simulink model "sampleModel1567_5_sub"  (R2023a)
settings: Solver=VariableStepAuto  StartTime=0.0  StopTime=10.0  RelTol=1e-3
libraries: hdlsllib x6
settings Model: Creator=user1  LastModifiedBy=user1

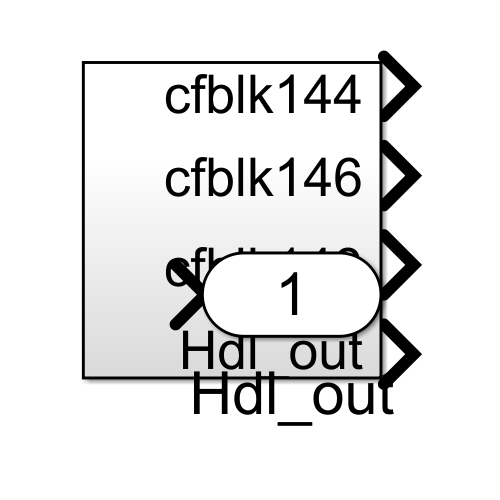
[thumbnail: Simulink's stored preview of the top-level diagram]
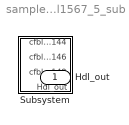
== system sampleModel1567_5_sub ==
  Subsystem : Subsystem
  Hdl_out : Outport  OutDataTypeStr=uint8

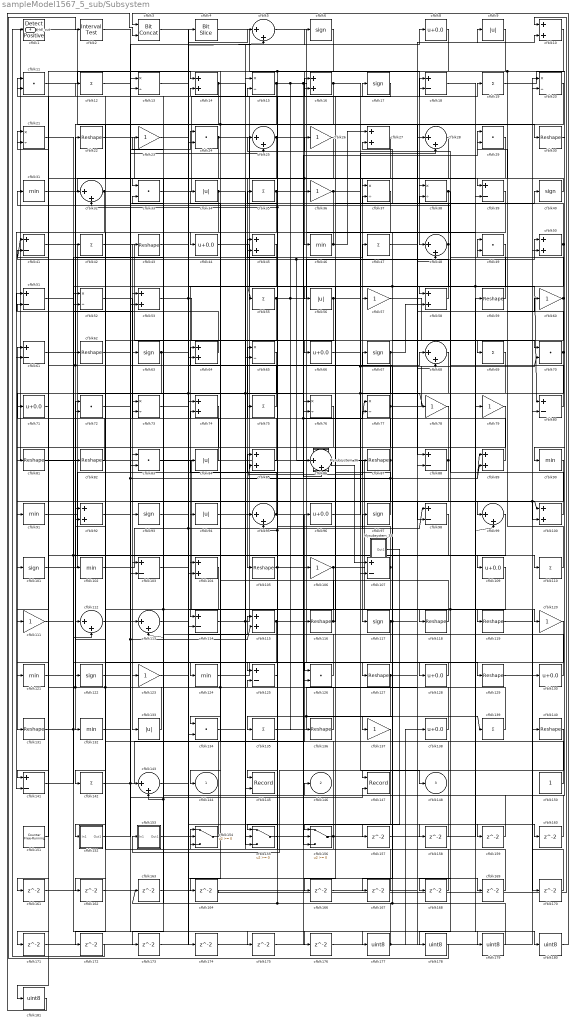
== system sampleModel1567_5_sub/Subsystem ==
  Mysubsystem_35 : Subsystem  TreatAsAtomicUnit=on  RTWFcnName=Mysubsystem_35
      settings: RTWFcnNameOpts=User specified  RTWFileNameOpts=Use function name
  Mysubsystem_36 : Subsystem  TreatAsAtomicUnit=on  RTWFcnName=Mysubsystem_36
      settings: RTWFcnNameOpts=User specified  RTWFileNameOpts=Use function name
  cfblk1 : hdlsllib/Logic and Bit Operations/Detect Rise Positive  vinit=0  OutDataTypeStr=uint8
  cfblk{10,14,16,27,45,50,53,58,64,74,85,89,92,100,104,115} (16 alike) : Sum  OutDataTypeStr=uint8
  cfblk{6,17,40,63,67,93,97,101,117,122} (10 alike) : Signum
  cfblk{31,46,90..91,102,121,124,132} (8 alike) : MinMax  OutDataTypeStr=uint8
  cfblk{18,39,41,51,61,80,88,98,103,107,114,125,141} (13 alike) : Sum  Inputs=+-  OutDataTypeStr=uint8
  cfblk{22,30,43,59,62,81..82,87,105,116,118..119,127,129,131,136,140} (17 alike) : Reshape
  cfblk{23,26,36,57,60,78..79,106,111,120,123,137} (12 alike) : Gain  OutDataTypeStr=uint8
  cfblk{8,44,66,71,96,109,128,130,138} (9 alike) : Bias  Bias=0.0  SaturateOnIntegerOverflow=off
  cfblk{11,24,29,33,49,70,72,83,126,134} (10 alike) : DotProduct  OutDataTypeStr=uint8
  cfblk{12,19,35,42,47,55,69,75,110,135,139,142} (12 alike) : Sum  Inputs=+  OutDataTypeStr=uint8
  cfblk{5,25,28,32,48,68,86,95,99,112..113,143} (12 alike) : Sum  Inputs=|++  OutDataTypeStr=uint8
  cfblk{13,15,20..21,37..38,52,65,73,76..77} (11 alike) : Product  Inputs=*/  OutDataTypeStr=uint8  RndMeth=Zero  SaturateOnIntegerOverflow=on
  cfblk{9,34,56,84,94,133} (6 alike) : Abs  OutDataTypeStr=uint8  SaturateOnIntegerOverflow=off
  cfblk145 : Record  FileSettingsInternal="{\"entries\":[{\"content\":{\"excelSettings\":{\"content\":{},\"type\":\"Streamout.ExcelSettings\"}},\"type\":\"Streamout.FileSettingStorage\",\"uuid\":\"\"}],\"packageUris\":[\"http:\\/\\/schema.mathworks.com\\/mf0\\/streamout_blocks\\/R2020a\"],\"version\":\"1.0\"}"  Layout=[1 1]  SignalsInternal="{\"entries\":[{\"content\":{\"signals\":[{\"content\":{\"blockPath\":[],\"dimensions\":[1],\"domain\":\"\",\"lineColor\":\"#a2142f\",\"plots\":[1],\"port\":1,\"signalID\":25340,\"signalName\":\"cfblk105\"},\"type\":\"RecordBlkView.Signal\",\"uuid\":\"\"},{\"content\":{\"blockPath\":[],\"dimensions\":[1],\"domain\":\"\",\"lineColor\":\"#139fff\",\"plots\":[1],\"port\":2,\"signalID\":25343,\"signalName\":\"cfblk109\"},\"type\":\"RecordBlkView.Signal\",\"uuid\":\"\"}]},\"type\":\"RecordBlkView.InputSignals\",\"uuid\":\"\"}],\"packageUris\":[\"http:\\/\\/schema.mathworks.com\\/mf0\\/streamout_blocks\\/R2020a\"],\"version\":\"1.0\"}"  VisualizationBindings="{\"xyplotplugin\":{\"info\":[{\"series\":[{\"bindingParametersList\":[{\"parameter\":\"X-Axis\",\"signalID\":25340,\"signalName\":\"cfblk105\"},{\"parameter\":\"Y-Axis\",\"signalID\":25343,\"signalName\":\"cfblk109\"}],\"seriesID\":58215}],\"subplotID\":1}]}}"  CompatibilityTag=XY  st=-1
  cfblk147 : Record  FileSettingsInternal="{\"entries\":[{\"content\":{\"excelSettings\":{\"content\":{},\"type\":\"Streamout.ExcelSettings\"}},\"type\":\"Streamout.FileSettingStorage\",\"uuid\":\"\"}],\"packageUris\":[\"http:\\/\\/schema.mathworks.com\\/mf0\\/streamout_blocks\\/R2020a\"],\"version\":\"1.0\"}"  Layout=[1 1]  SignalsInternal="{\"entries\":[{\"content\":{\"signals\":[{\"content\":{\"blockPath\":[],\"dimensions\":[1],\"domain\":\"\",\"lineColor\":\"#a2142f\",\"plots\":[1],\"port\":1,\"signalID\":25332,\"signalName\":\"cfblk117\"},\"type\":\"RecordBlkView.Signal\",\"uuid\":\"\"},{\"content\":{\"blockPath\":[],\"dimensions\":[1],\"domain\":\"\",\"lineColor\":\"#139fff\",\"plots\":[1],\"port\":2,\"signalID\":25335,\"signalName\":\"cfblk142\"},\"type\":\"RecordBlkView.Signal\",\"uuid\":\"\"}]},\"type\":\"RecordBlkView.InputSignals\",\"uuid\":\"\"}],\"packageUris\":[\"http:\\/\\/schema.mathworks.com\\/mf0\\/streamout_blocks\\/R2020a\"],\"version\":\"1.0\"}"  VisualizationBindings="{\"xyplotplugin\":{\"info\":[{\"series\":[{\"bindingParametersList\":[{\"parameter\":\"X-Axis\",\"signalID\":25332,\"signalName\":\"cfblk117\"},{\"parameter\":\"Y-Axis\",\"signalID\":25335,\"signalName\":\"cfblk142\"}],\"seriesID\":62710}],\"subplotID\":1}]}}"  CompatibilityTag=XY  st=-1
  cfblk150 : Constant  OutDataTypeStr=uint8  SampleTime=-1
  cfblk151 : hdlsllib/Sources/Counter Free-Running  NumBits=16  tsamp=-1
  cfblk152 : Subsystem
      settings: LibrarySourceBlock=|
      | hdlsllib/Ports &
      | Subsystems/Subsystem
  cfblk153 : Subsystem
      settings: LibrarySourceBlock=|
      | hdlsllib/Ports &
      | Subsystems/Subsystem
  cfblk154 : Switch  OutDataTypeStr=uint8  SaturateOnIntegerOverflow=off  InputSameDT=off
  cfblk155 : Switch  OutDataTypeStr=uint8  SaturateOnIntegerOverflow=off  InputSameDT=off
  cfblk156 : Switch  OutDataTypeStr=uint8  SaturateOnIntegerOverflow=off  InputSameDT=off
  cfblk{157..164,166..176} (19 alike) : Delay  SampleTime=1
  cfblk{177..181} (5 alike) : DataTypeConversion  OutDataTypeStr=uint8  SaturateOnIntegerOverflow=off  RndMeth=Floor
  cfblk2 : hdlsllib/Logic and Bit Operations/Interval Test  IntervalClosedRight=on  uplimit=0.5  IntervalClosedLeft=on  lowlimit=-0.5  OutDataTypeStr=uint8
  cfblk3 : hdlsllib/Logic and Bit Operations/Bit Concat  numInputs=2
  cfblk4 : hdlsllib/Logic and Bit Operations/Bit Slice  lidx=7  ridx=0
  cfblk144 : Outport  OutDataTypeStr=uint8  VectorParamsAs1DForOutWhenUnconnected=off
  cfblk146 : Outport  Port=2  OutDataTypeStr=uint8  VectorParamsAs1DForOutWhenUnconnected=off
  cfblk148 : Outport  Port=3  OutDataTypeStr=uint8  VectorParamsAs1DForOutWhenUnconnected=off
  Hdl_out : Outport  Port=4  OutDataTypeStr=uint8
  wires:
  cfblk40/1 -> cfblk33/1
  cfblk20/1 -> cfblk132/1
  cfblk56/1 -> cfblk58/1, cfblk142/1
  cfblk75/1 -> cfblk41/2, cfblk22/1
  cfblk107/1 -> cfblk133/1, cfblk32/2, cfblk11/2
  cfblk127/1 -> cfblk60/1, cfblk154/1
  cfblk63/1 -> cfblk5/1, cfblk131/1
  cfblk41/1 -> cfblk110/1
  cfblk140/1 -> cfblk153/1(In1)
  cfblk33/1 -> cfblk17/1
  cfblk153/1(Out1) -> cfblk98/1, cfblk4/1
  cfblk91/1 -> cfblk109/1
  cfblk44/1 -> cfblk99/2, cfblk80/1
  cfblk35/1 -> cfblk141/2, cfblk128/1
  cfblk114/1 -> cfblk8/1, cfblk19/1
  cfblk67/1 -> cfblk58/2, cfblk164/1, cfblk155/3
  cfblk59/1 -> cfblk31/1
  cfblk87/1 -> Hdl_out/1, cfblk12/1, cfblk114/1
  cfblk27/1 -> cfblk105/1
  cfblk22/1 -> cfblk117/1
  cfblk83/1 -> cfblk120/1
  cfblk136/1 -> cfblk11/1, cfblk72/1
  cfblk79/1 -> cfblk144/1
  cfblk84/1 -> cfblk61/1
  cfblk126/1 -> cfblk95/2, cfblk35/1
  cfblk99/1 -> cfblk122/1
  cfblk90/1 -> cfblk123/1
  cfblk42/1 -> cfblk69/1
  cfblk48/1 -> cfblk16/1, cfblk55/1, cfblk137/1
  cfblk8/1 -> cfblk46/1
  cfblk122/1 -> cfblk115/2, cfblk89/1, cfblk45/1
  cfblk5/1 -> cfblk79/1
  cfblk106/1 -> cfblk155/2, cfblk119/1
  cfblk69/1 -> cfblk93/1
  cfblk12/1 -> cfblk113/1
  cfblk19/1 -> cfblk146/1
  cfblk141/1 -> cfblk52/1
  cfblk15/1 -> cfblk106/1, cfblk39/2, cfblk30/1, cfblk32/1, cfblk124/1
  cfblk85/1 -> cfblk65/1
  cfblk142/1 -> cfblk147/2, cfblk96/1
  cfblk46/1 -> cfblk27/1, cfblk44/1
  cfblk50/1 -> cfblk27/2, cfblk94/1
  cfblk53/1 -> cfblk5/2, cfblk66/1
  cfblk81/1 -> cfblk82/1
  cfblk25/1 -> cfblk171/1, cfblk37/1
  cfblk86/1 -> cfblk140/1
  cfblk29/1 -> cfblk36/1, cfblk173/1, cfblk143/2
  cfblk89/1 -> cfblk43/1
  cfblk131/1 -> cfblk176/1, cfblk47/1
  cfblk113/1 -> cfblk74/1
  cfblk130/1 -> cfblk42/1
  cfblk150/1 -> cfblk74/2
  cfblk4/1 -> cfblk48/1
  cfblk57/1 -> cfblk70/1
  cfblk9/1 -> cfblk121/1
  cfblk32/1 -> cfblk61/2, cfblk100/2, cfblk100/1
  cfblk92/1 -> cfblk40/1
  cfblk151/1 -> cfblk71/1
  cfblk52/1 -> cfblk73/1
  cfblk82/1 -> cfblk72/2
  cfblk30/1 -> cfblk90/1
  cfblk34/1 -> cfblk158/1, cfblk83/2
  cfblk55/1 -> cfblk65/2, cfblk136/1, cfblk50/1
  cfblk58/1 -> cfblk41/1, Mysubsystem_36/1(In1)
  cfblk101/1 -> cfblk37/2, cfblk77/1
  cfblk45/1 -> cfblk52/2
  cfblk72/1 -> cfblk143/1
  cfblk11/1 -> cfblk14/1
  cfblk66/1 -> cfblk70/2, cfblk107/2
  cfblk10/1 -> cfblk39/1, cfblk125/1, cfblk104/1
  cfblk80/1 -> cfblk26/1
  cfblk26/1 -> cfblk63/1
  cfblk71/1 -> cfblk141/1
  cfblk17/1 -> cfblk14/2
  cfblk31/1 -> cfblk38/1
  cfblk133/1 -> cfblk92/1, cfblk51/2
  cfblk70/1 -> cfblk29/2, cfblk134/1
  cfblk78/1 -> cfblk104/2
  cfblk116/1 -> cfblk16/2, cfblk64/1
  cfblk1/1 -> cfblk88/1
  cfblk38/1 -> cfblk168/1, cfblk91/1
  cfblk95/1 -> cfblk84/1, cfblk156/2
  cfblk124/1 -> cfblk126/1
  cfblk125/1 -> cfblk15/2
  cfblk94/1 -> cfblk87/1
  cfblk61/1 -> cfblk154/2
  cfblk117/1 -> cfblk156/3, cfblk10/2, cfblk147/1
  cfblk76/1 -> cfblk135/1
  cfblk102/1 -> cfblk97/1
  cfblk103/1 -> cfblk68/1
  cfblk110/1 -> cfblk49/1
  cfblk156/1 -> cfblk92/2, cfblk154/3, cfblk59/1
  cfblk105/1 -> cfblk116/1, cfblk145/1
  cfblk39/1 -> cfblk57/1
  cfblk68/1 -> cfblk111/1
  cfblk28/1 -> cfblk75/1
  cfblk88/1 -> cfblk81/1, cfblk101/1
  cfblk132/1 -> cfblk24/1
  cfblk123/1 -> cfblk115/1
  cfblk134/1 -> cfblk18/1
  cfblk47/1 -> cfblk9/1
  cfblk115/1 -> cfblk29/1, cfblk152/1(In1)
  cfblk24/1 -> cfblk103/1, cfblk86/2
  cfblk62/1 -> cfblk6/1
  cfblk129/1 -> cfblk130/1
  cfblk109/1 -> cfblk178/1, cfblk145/2
  cfblk51/1 -> cfblk112/2
  cfblk121/1 -> cfblk53/1
  cfblk97/1 -> cfblk85/2, cfblk25/1
  cfblk100/1 -> cfblk38/2
  cfblk96/1 -> cfblk28/2
  cfblk152/1(Out1) -> cfblk25/2
  cfblk64/1 -> cfblk33/2
  cfblk154/1 -> cfblk62/1
  cfblk139/1 -> cfblk21/2, cfblk34/1
  cfblk60/1 -> cfblk167/1, cfblk49/2
  cfblk13/1 -> cfblk118/1, cfblk76/2
  cfblk37/1 -> cfblk95/1
  cfblk65/1 -> cfblk83/1
  cfblk77/1 -> cfblk21/1, cfblk102/1, cfblk20/2
  cfblk112/1 -> cfblk89/2, cfblk13/2
  cfblk3/1 -> cfblk179/1
  cfblk104/1 -> cfblk162/1, cfblk113/2
  cfblk21/1 -> cfblk103/2, cfblk129/1
  cfblk118/1 -> cfblk85/1
  cfblk43/1 -> cfblk56/1
  cfblk135/1 -> cfblk68/2, cfblk139/1
  cfblk2/1 -> cfblk177/1
  cfblk138/1 -> cfblk23/1
  cfblk14/1 -> cfblk134/2, cfblk18/2
  cfblk120/1 -> cfblk155/1
  cfblk36/1 -> cfblk172/1, cfblk98/2
  cfblk16/1 -> cfblk53/2, cfblk148/1, cfblk78/1
  cfblk93/1 -> cfblk99/1
  cfblk128/1 -> cfblk127/1
  cfblk6/1 -> cfblk64/2
  cfblk137/1 -> cfblk157/1
  cfblk157/1 -> cfblk77/2
  cfblk158/1 -> cfblk76/1
  cfblk155/1 -> cfblk159/1
  cfblk159/1 -> cfblk51/1
  cfblk73/1 -> cfblk160/1
  cfblk160/1 -> cfblk13/1
  cfblk74/1 -> cfblk161/1
  cfblk161/1 -> cfblk88/2
  cfblk162/1 -> cfblk114/2
  cfblk163/1 -> cfblk126/2
  cfblk164/1 -> cfblk10/1
  cfblk49/1 -> cfblk166/1
  cfblk166/1 -> cfblk28/1
  cfblk167/1 -> cfblk125/2
  cfblk168/1 -> cfblk112/1
  cfblk23/1 -> cfblk169/1
  cfblk169/1 -> cfblk15/1
  cfblk119/1 -> cfblk170/1
  cfblk170/1 -> cfblk20/1
  cfblk171/1 -> cfblk48/2
  cfblk172/1 -> cfblk1/1
  cfblk173/1 -> cfblk24/2
  cfblk143/1 -> cfblk174/1
  cfblk174/1 -> cfblk86/1
  cfblk111/1 -> cfblk175/1
  cfblk175/1 -> cfblk80/2
  cfblk176/1 -> cfblk50/2
  cfblk177/1 -> cfblk138/1, cfblk73/2, cfblk45/2
  cfblk178/1 -> cfblk2/1
  cfblk179/1 -> cfblk67/1, cfblk163/1
  cfblk18/1 -> cfblk180/1
  cfblk180/1 -> cfblk3/1
  cfblk98/1 -> cfblk181/1
  cfblk181/1 -> cfblk3/2
  Mysubsystem_35/1(Out1) -> cfblk156/1
  Mysubsystem_36/1(Out1) -> cfblk107/1

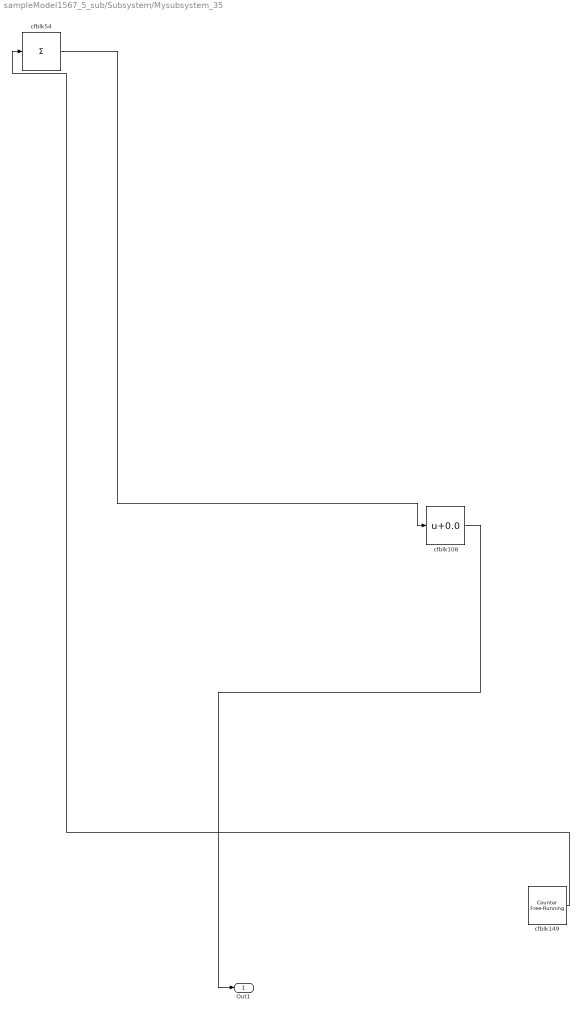
== system sampleModel1567_5_sub/Subsystem/Mysubsystem_35 ==
  cfblk108 : Bias  Bias=0.0  SaturateOnIntegerOverflow=off
  cfblk149 : hdlsllib/Sources/Counter Free-Running  NumBits=16  tsamp=-1
  cfblk54 : Sum  Inputs=+
  Out1 : Outport
  wires:
  cfblk149/1 -> cfblk54/1
  cfblk108/1 -> Out1/1
  cfblk54/1 -> cfblk108/1

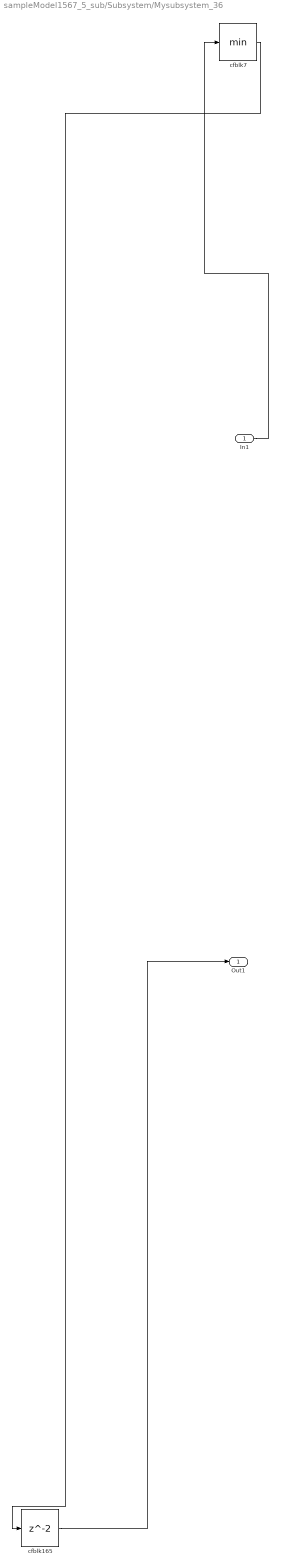
== system sampleModel1567_5_sub/Subsystem/Mysubsystem_36 ==
  In1 : Inport
  cfblk165 : Delay  SampleTime=1
  cfblk7 : MinMax
  Out1 : Outport
  wires:
  In1/1 -> cfblk7/1
  cfblk165/1 -> Out1/1
  cfblk7/1 -> cfblk165/1

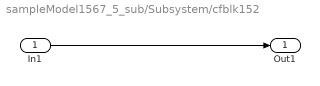
== system sampleModel1567_5_sub/Subsystem/cfblk152 ==
  In1 : Inport
  Out1 : Outport
  wires:
  In1/1 -> Out1/1

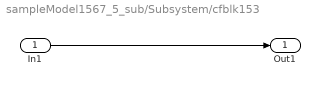
== system sampleModel1567_5_sub/Subsystem/cfblk153 ==
  In1 : Inport
  Out1 : Outport
  wires:
  In1/1 -> Out1/1
